simulink model "SystemDiffEquation"  (R2020a)
settings: Solver=VariableStepAuto  StartTime=0.0  StopTime=10.0  RelTol=1e-3
settings Model: Creator=Mohammad  LastModifiedBy=Mohammad

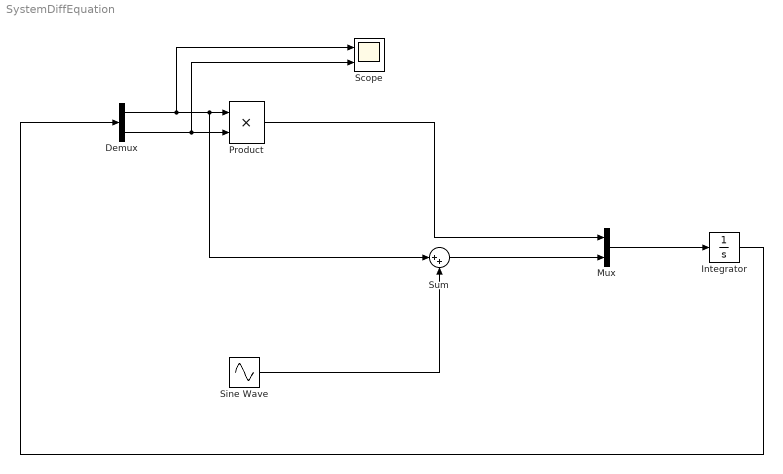
== system SystemDiffEquation ==
  Demux : Demux  Outputs=2
  Integrator : Integrator  InitialCondition=[1e-6 0.001]
  Mux : Mux  Inputs=2
  Product : Product
  Scope : Scope  NumInputPorts=2
  Sine Wave : Sin  SampleTime=0
  Sum : Sum  Inputs=|++
  wires:
  Mux/1 -> Integrator/1
  Sum/1 -> Mux/2
  Demux/2 -> Scope/2, Product/2
  Demux/1 -> Scope/1, Sum/1, Product/1
  Product/1 -> Mux/1
  Integrator/1 -> Demux/1
  Sine Wave/1 -> Sum/2
